simulink model "RL_vehicle_dynamic_model02"  (R2019b)
settings: Solver=ode45  StartTime=0.0  StopTime=60  RelTol=1e-3
model workspace (MAT data in the model file):
  kappar = [0 0 0 0 0 0 0 0 0 0 0 0 ... (4802 elements, 1x4802)]
  thetar = [0 0 0 0 0 0 0 0 0 0 0 0 ... (4802 elements, 1x4802)]
  xr = [0.0501253132832 0.100250626566 0.15037593985 0.200501253133 0.250626566416 0.300751879699 0.350877192982 0.401002506266 0.451127819549 0.501253132832 0.551378446115 0.601503759398 ... (4802 elements, 1x4802)]
  yr = [0 0 0 0 0 0 0 0 0 0 0 0 ... (4802 elements, 1x4802)]
libraries: simulink x3, rllib x1
(part 2 of 2)

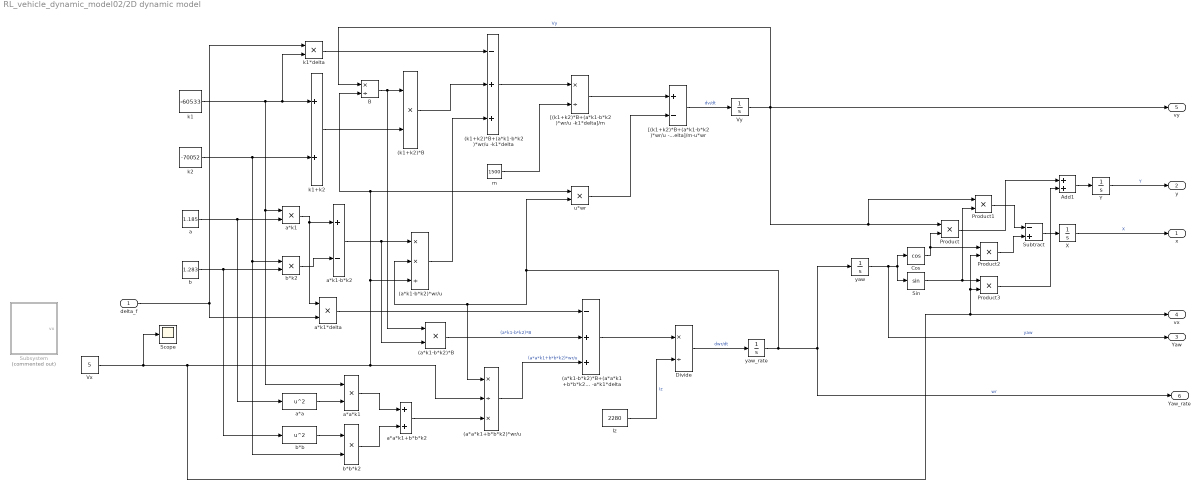
== system RL_vehicle_dynamic_model02/2D dynamic model ==
  delta_f : Inport
  (a*a*k1+b*b*k2)*wr/u : Product  Inputs=*/*
  (a*k1-b*k2)*B : Product
  (a*k1-b*k2)*B+(a*a*k1+b*b*k2)*wr/u -a*k1*delta : Sum  Inputs=-++
  (a*k1-b*k2)*wr/u : Product  Inputs=**/
  (k1+k2)*B : Product
  (k1+k2)*B+(a*k1-b*k2)*wr/u -k1*delta : Sum  Inputs=-++
  Add1 : Sum
  B : Product  Inputs=*/
  Cos : Trigonometry  Operator=cos
  Divide : Product  Inputs=*/
  Iz : Constant  Value=2280
  Product{,1..3} (4 alike) : Product
  Scope : Scope
  Sin : Trigonometry
  Subsystem : Subsystem  Commented=on
  Subtract : Sum  Inputs=-+
  Vx : Constant  Value=5
  Vy : Integrator
  X : Integrator
  Y : Integrator
  "[(k1+k2)*B+(a*k1-b*k2)*wr/u -k1*delta]/m" : Product  Inputs=*/
  "[(k1+k2)*B+(a*k1-b*k2)*wr/u -k1*delta]/m-u*wr" : Sum  Inputs=+-
  a : Constant  Value=1.185
  a*a : Fcn  Expr=u^2
  a*a*k1 : Product
  a*a*k1+b*b*k2 : Sum
  a*k1 : Product
  a*k1*delta : Product
  a*k1-b*k2 : Sum  Inputs=+-
  b : Constant  Value=1.283
  b*b : Fcn  Expr=u^2
  b*b*k2 : Product
  b*k2 : Product
  k1 : Constant  Value=-60533
  k1*delta : Product
  k1+k2 : Sum
  k2 : Constant  Value=-70052
  m : Constant  Value=1500
  u*wr : Product
  yaw : Integrator
  yaw_rate : Integrator
  x : Outport  VectorParamsAs1DForOutWhenUnconnected=off
  y : Outport  Port=2  VectorParamsAs1DForOutWhenUnconnected=off
  Yaw : Outport  Port=3  VectorParamsAs1DForOutWhenUnconnected=off
  vx : Outport  Port=4  VectorParamsAs1DForOutWhenUnconnected=off
  vy : Outport  Port=5  VectorParamsAs1DForOutWhenUnconnected=off
  Yaw_rate : Outport  Port=6  VectorParamsAs1DForOutWhenUnconnected=off
  wires:
  (a*a*k1+b*b*k2)*wr/u/1 -> (a*k1-b*k2)*B+(a*a*k1+b*b*k2)*wr/u -a*k1*delta/3  "(a*a*k1+b*b*k2)*wr/u"
  b/1 -> b*k2/2, b*b/1
  (a*k1-b*k2)*B+(a*a*k1+b*b*k2)*wr/u -a*k1*delta/1 -> Divide/1
  k1+k2/1 -> (k1+k2)*B/2
  yaw/1 -> Yaw/1, Cos/1, Sin/1  "yaw"
  k1/1 -> k1*delta/2, k1+k2/1, a*a*k1/1, a*k1/1
  k2/1 -> k1+k2/2, b*b*k2/2, b*k2/1
  b*b/1 -> b*b*k2/1
  Product2/1 -> Subtract/2
  B/1 -> (a*k1-b*k2)*B/1, (k1+k2)*B/1
  Add1/1 -> Y/1
  Sin/1 -> Product3/1, Product1/2
  "[(k1+k2)*B+(a*k1-b*k2)*wr/u -k1*delta]/m"/1 -> "[(k1+k2)*B+(a*k1-b*k2)*wr/u -k1*delta]/m-u*wr"/1
  yaw_rate/1 -> (a*k1-b*k2)*wr/u/2, (a*a*k1+b*b*k2)*wr/u/1, u*wr/2, yaw/1, Yaw_rate/1  "wr"
  a/1 -> a*k1/2, a*a/1
  Product/1 -> Add1/1
  a*k1-b*k2/1 -> (a*k1-b*k2)*B/2, (a*k1-b*k2)*wr/u/1
  Product3/1 -> Add1/2
  b*b*k2/1 -> a*a*k1+b*b*k2/2
  Vy/1 -> vy/1, Product/1, Product1/1, B/1  "Vy"
  a*a*k1/1 -> a*a*k1+b*b*k2/1
  "[(k1+k2)*B+(a*k1-b*k2)*wr/u -k1*delta]/m-u*wr"/1 -> Vy/1  "dv/dt"
  u*wr/1 -> "[(k1+k2)*B+(a*k1-b*k2)*wr/u -k1*delta]/m-u*wr"/2
  (k1+k2)*B+(a*k1-b*k2)*wr/u -k1*delta/1 -> "[(k1+k2)*B+(a*k1-b*k2)*wr/u -k1*delta]/m"/1
  a*k1/1 -> a*k1*delta/1, a*k1-b*k2/1
  a*a*k1+b*b*k2/1 -> (a*a*k1+b*b*k2)*wr/u/3
  Iz/1 -> Divide/2  "Iz"
  (a*k1-b*k2)*B/1 -> (a*k1-b*k2)*B+(a*a*k1+b*b*k2)*wr/u -a*k1*delta/2  "(a*k1-b*k2)*B"
  (a*k1-b*k2)*wr/u/1 -> (k1+k2)*B+(a*k1-b*k2)*wr/u -k1*delta/3
  delta_f/1 -> a*k1*delta/2, k1*delta/1
  a*a/1 -> a*a*k1/2
  Y/1 -> y/1  "Y"
  (k1+k2)*B/1 -> (k1+k2)*B+(a*k1-b*k2)*wr/u -k1*delta/2
  Cos/1 -> Product2/1, Product/2
  a*k1*delta/1 -> (a*k1-b*k2)*B+(a*a*k1+b*b*k2)*wr/u -a*k1*delta/1
  b*k2/1 -> a*k1-b*k2/2
  k1*delta/1 -> (k1+k2)*B+(a*k1-b*k2)*wr/u -k1*delta/1
  m/1 -> "[(k1+k2)*B+(a*k1-b*k2)*wr/u -k1*delta]/m"/2
  Divide/1 -> yaw_rate/1  "dwr/dt"
  Subtract/1 -> X/1
  Product1/1 -> Subtract/1
  X/1 -> x/1  "X"
  Vx/1 -> Scope/1, vx/1, Product3/2, Product2/2, B/2, u*wr/1, (a*k1-b*k2)*wr/u/3, (a*a*k1+b*b*k2)*wr/u/2

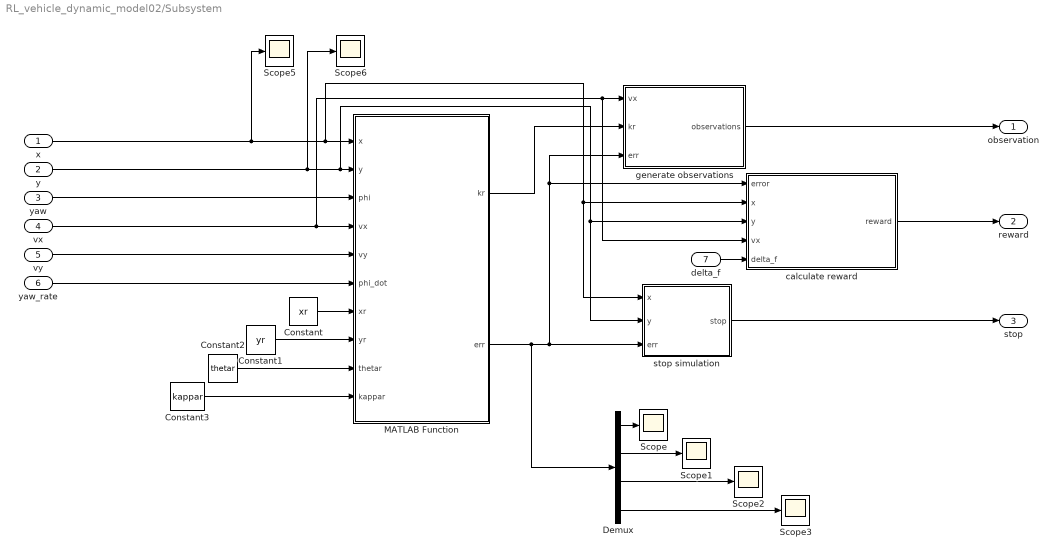
== system RL_vehicle_dynamic_model02/Subsystem ==
  x : Inport
  y : Inport  Port=2
  yaw : Inport  Port=3
  vx : Inport  Port=4
  vy : Inport  Port=5
  yaw_rate : Inport  Port=6
  delta_f : Inport  Port=7
  Constant : Constant  Value=xr
  Constant1 : Constant  Value=yr
  Constant2 : Constant  Value=thetar
  Constant3 : Constant  Value=kappar
  Demux : Demux
  MATLAB Function : MATLAB Function  TreatAsAtomicUnit=on
  Scope{,1..3,5..6} (6 alike) : Scope
  calculate reward : Subsystem
  generate observations : Subsystem
  stop simulation : Subsystem
  observation : Outport
  reward : Outport  Port=2
  stop : Outport  Port=3
  wires:
  y/1 -> Scope6/1, stop simulation/2(y), calculate reward/3(y), MATLAB Function/2(y)
  Demux/3 -> Scope2/1
  vx/1 -> calculate reward/4(vx), generate observations/1(vx), MATLAB Function/4(vx)
  stop simulation/1(stop) -> stop/1
  Demux/4 -> Scope3/1
  Constant/1 -> MATLAB Function/7(xr)
  Demux/2 -> Scope1/1
  MATLAB Function/2(err) -> stop simulation/3(err), generate observations/3(err), calculate reward/1(error), Demux/1
  yaw/1 -> MATLAB Function/3(phi)
  x/1 -> Scope5/1, MATLAB Function/1(x), stop simulation/1(x), calculate reward/2(x)
  MATLAB Function/1(kr) -> generate observations/2(kr)
  Constant3/1 -> MATLAB Function/10(kappar)
  Constant2/1 -> MATLAB Function/9(thetar)
  Constant1/1 -> MATLAB Function/8(yr)
  Demux/1 -> Scope/1
  calculate reward/1(reward) -> reward/1
  vy/1 -> MATLAB Function/5(vy)
  yaw_rate/1 -> MATLAB Function/6(phi_dot)
  generate observations/1(observations) -> observation/1
  delta_f/1 -> calculate reward/5(delta_f)

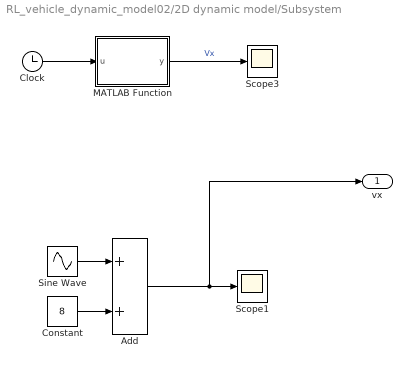
== system RL_vehicle_dynamic_model02/2D dynamic model/Subsystem ==
  Add : Sum
  Clock : Clock
  Constant : Constant  Value=8
  MATLAB Function : MATLAB Function  TreatAsAtomicUnit=on
  Scope1 : Scope
  Scope3 : Scope
  Sine Wave : Sin  Amplitude=5  Frequency=0.05*pi  SampleTime=0.1
  vx : Outport
  wires:
  MATLAB Function/1(y) -> Scope3/1  "Vx"
  Sine Wave/1 -> Add/1
  Clock/1 -> MATLAB Function/1(u)
  Add/1 -> vx/1, Scope1/1
  Constant/1 -> Add/2

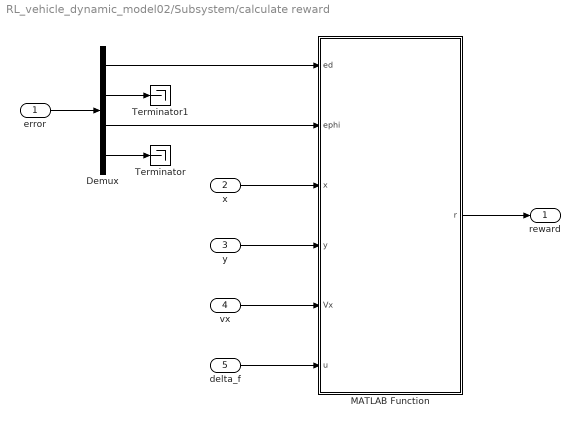
== system RL_vehicle_dynamic_model02/Subsystem/calculate reward ==
  error : Inport
  x : Inport  Port=2
  y : Inport  Port=3
  vx : Inport  Port=4
  delta_f : Inport  Port=5
  Demux : Demux
  MATLAB Function : MATLAB Function  TreatAsAtomicUnit=on
  Terminator : Terminator
  Terminator1 : Terminator
  reward : Outport  VectorParamsAs1DForOutWhenUnconnected=off
  wires:
  error/1 -> Demux/1
  MATLAB Function/1(r) -> reward/1
  Demux/4 -> Terminator/1
  Demux/1 -> MATLAB Function/1(ed)
  Demux/3 -> MATLAB Function/2(ephi)
  Demux/2 -> Terminator1/1
  x/1 -> MATLAB Function/3(x)
  y/1 -> MATLAB Function/4(y)
  vx/1 -> MATLAB Function/5(Vx)
  delta_f/1 -> MATLAB Function/6(u)

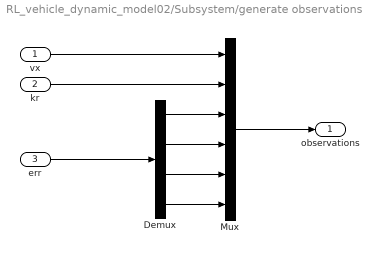
== system RL_vehicle_dynamic_model02/Subsystem/generate observations ==
  vx : Inport
  kr : Inport  Port=2
  err : Inport  Port=3
  Demux : Demux
  Mux : Mux  Inputs=6
  observations : Outport
  wires:
  vx/1 -> Mux/1
  Mux/1 -> observations/1
  kr/1 -> Mux/2
  err/1 -> Demux/1
  Demux/1 -> Mux/3
  Demux/2 -> Mux/4
  Demux/3 -> Mux/5
  Demux/4 -> Mux/6

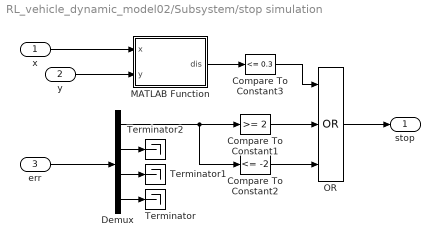
== system RL_vehicle_dynamic_model02/Subsystem/stop simulation ==
  x : Inport
  y : Inport  Port=2
  err : Inport  Port=3
  Compare To Constant1 : simulink/Logic and Bit Operations/Compare To Constant  relop=>=  const=2  OutDataTypeStr=boolean
  Compare To Constant2 : simulink/Logic and Bit Operations/Compare To Constant  relop=<=  const=-2  OutDataTypeStr=boolean
  Compare To Constant3 : simulink/Logic and Bit Operations/Compare To Constant  relop=<=  const=0.3  OutDataTypeStr=boolean
  Demux : Demux
  MATLAB Function : MATLAB Function  TreatAsAtomicUnit=on
  OR : Logic  Operator=OR  Inputs=3  IconShape=distinctive  AllPortsSameDT=off  OutDataTypeStr=boolean
  Terminator : Terminator
  Terminator1 : Terminator
  Terminator2 : Terminator
  stop : Outport  VectorParamsAs1DForOutWhenUnconnected=off
  wires:
  Compare To Constant2/1 -> OR/3
  Compare To Constant1/1 -> OR/2
  OR/1 -> stop/1
  err/1 -> Demux/1
  Demux/4 -> Terminator/1
  Demux/1 -> Compare To Constant1/1, Compare To Constant2/1
  Demux/3 -> Terminator1/1
  Demux/2 -> Terminator2/1
  x/1 -> MATLAB Function/1(x)
  y/1 -> MATLAB Function/2(y)
  MATLAB Function/1(dis) -> Compare To Constant3/1
  Compare To Constant3/1 -> OR/1

== matlab function RL_vehicle_dynamic_model02/Subsystem/calculate reward/MATLAB Function ==
  data: ed input; r output; ephi input; x input; y input; Vx input; u input
function r = fcn(ed, ephi, x, y, Vx, u)

r1 = -(ed*ed + 0.5*ephi*ephi + 0.1*u*u); % 限制转向角大小

if abs(ed) <= 0.2
    H = 2;
elseif abs(ed) <= 0.5
    H = 1;
else
    H = 0;
end

if abs(ed) >= 2
    F = 2;
elseif abs(ed) >= 1
    F = 1;
else
    F = 0;
end

if abs(ephi) <= 5/180*pi
    M = 2;
elseif abs(ephi) <= 10/180*pi
    M = 1;
else
    M = 0;
end

if abs(ephi) >= 20/180*pi
    N = 1;
else
    N = 0;
end
r2 = -1*F + 1*H + 1*M - 1*N;

x0 = 240;
y0 = 0;
dis = ((x-x0)^2 + (y-y0)^2)^0.5;
if dis <= 0.2
    r3 = 100;
else
    r3 = 0;
end

r = (r1 + r2) * Vx/5;

== matlab function RL_vehicle_dynamic_model02/Subsystem/MATLAB Function ==
  data: x input; kr output; y input; phi input; vx input; vy input; phi_dot input; xr input; yr input; thetar input; kappar input; err output
function [kr,err] = fcn(x,y,phi,vx,vy,phi_dot,xr,yr,thetar,kappar)

n=length(xr);
d_min=(x-xr(1))^2+(y-yr(1))^2;
min=1;
for i=1:n
    d=(x-xr(i))^2+(y-yr(i))^2;
    if d<d_min
        d_min=d;
        min=i;
    end
end
dmin=min;
tor=[cos(thetar(dmin));sin(thetar(dmin))];
nor=[-sin(thetar(dmin));cos(thetar(dmin))];
d_err=[x-xr(dmin);y-yr(dmin)];
ed=nor'*d_err;
es=tor'*d_err;
%projection_point_thetar=thetar(dmin);   %apollo
projection_point_thetar=thetar(dmin)+kappar(dmin)*es;
ed_dot=vy*cos(phi-projection_point_thetar)+vx*sin(phi-projection_point_thetar);
ephi=sin(phi-projection_point_thetar);
s_dot=vx*cos(phi-projection_point_thetar)-vy*sin(phi-projection_point_thetar);
s_dot=s_dot/(1-kappar(dmin)*ed);
ephi_dot=phi_dot-kappar(dmin)*s_dot;
kr=kappar(dmin);
err=[ed;ed_dot;ephi;ephi_dot];
end

== matlab function RL_vehicle_dynamic_model02/Subsystem/stop simulation/MATLAB Function ==
  data: x input; dis output; y input
function dis = fcn(x, y)

x0 = 240;
y0 = 0;
dis = ((x-x0)^2 + (y-y0)^2)^0.5;

== matlab function RL_vehicle_dynamic_model02/2D dynamic model/Subsystem/MATLAB Function ==
  data: u input; y output
function y = fcn(u)

if u <= 25
    y = 5+0.2*u;
else
    y = 10;
end
